simulink model "pdctrl"  (R2024b)
settings: Solver=VariableStepAuto  StartTime=0.0  StopTime=10.0  RelTol=1e-3
libraries: slpidlib x1
settings Model: Creator=Dell  LastModifiedBy=Dell

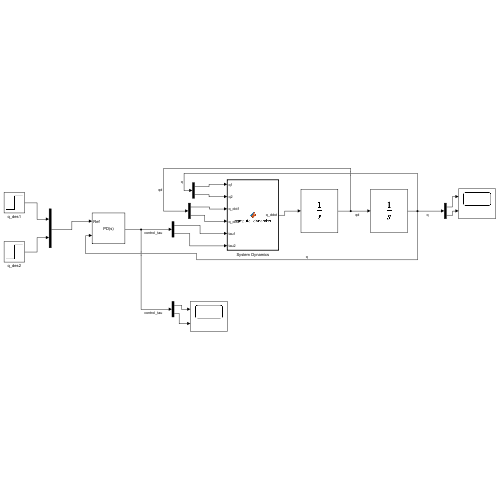
[thumbnail: Simulink's stored preview of the top-level diagram]
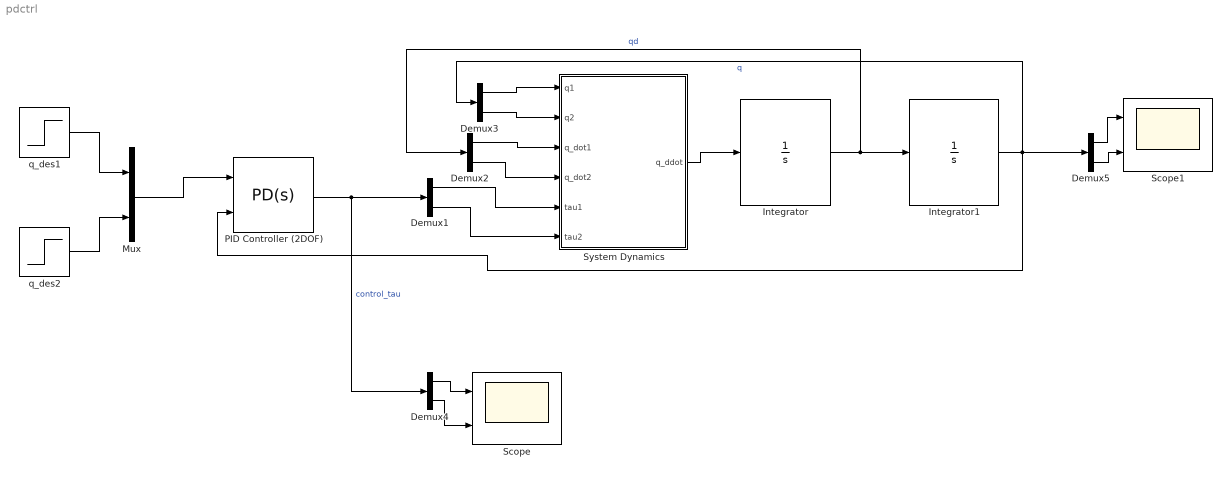
== system pdctrl ==
  Demux{1..5} (5 alike) : Demux  Outputs=2
  Integrator : Integrator  InitialCondition=[0;0]
  Integrator1 : Integrator  InitialCondition=[0, 0]
  Mux : Mux  Inputs=2
  PID Controller (2DOF) : slpidlib/PID Controller (2DOF)  Controller=PD  Form=Parallel  TimeDomain=Continuous-time  UseExternalTs=off  SampleTime=-1  IntegratorMethod=Forward Euler  FilterMethod=Forward Euler  ControllerParametersSource=internal  P=2000  I=0  UseKiTs=off  D=100  UseExternalDerivativeSource=off  N=100  UseFilter=on  b=1  c=1  TunerSelectOption=Transfer Function Based (PID Tuner App)  InitialConditionSource=internal  InitialConditionForIntegrator=0  InitialConditionForFilter=0  DifferentiatorICPrevScaledInput=0  ExternalReset=none  TrackingMode=off  Kt=1  LimitOutput=off  SatLimitsSource=internal  UpperSaturationLimit=inf  LowerSaturationLimit=-inf  LinearizeAsGain=on  AntiWindupMode=none  Kb=1  LimitIntegrator=off  UpperIntegratorSaturationLimit=inf  LowerIntegratorSaturationLimit=-inf  POutMin=[]  POutMax=[]  IOutMin=[]  IOutMax=[]  DOutMin=[]  DOutMax=[]  NOutMin=[]  NOutMax=[]  bOutMin=[]  bOutMax=[]  cOutMin=[]  cOutMax=[]  SumOutMin=[]  SumOutMax=[]  SaturationOutMin=[]  SaturationOutMax=[]  PParamMin=[]  PParamMax=[]  IParamMin=[]  IParamMax=[]  DParamMin=[]  DParamMax=[]  NParamMin=[]  NParamMax=[]  bParamMin=[]  bParamMax=[]  cParamMin=[]  cParamMax=[]  KbParamMin=[]  KbParamMax=[]  KtParamMin=[]  KtParamMax=[]  KbOutMin=[]  KbOutMax=[]  KtOutMin=[]  KtOutMax=[]  IntegratorOutMin=[]  IntegratorOutMax=[]  FilterOutMin=[]  FilterOutMax=[]  SumI1OutMin=[]  SumI1OutMax=[]  SumI2OutMin=[]  SumI2OutMax=[]  SumI3OutMin=[]  SumI3OutMax=[]  SumI4OutMin=[]  SumI4OutMax=[]  SumDOutMin=[]  SumDOutMax=[]  Sum1OutMin=[]  Sum1OutMax=[]  Sum2OutMin=[]  Sum2OutMax=[]  Sum3OutMin=[]  Sum3OutMax=[]  DifferentiatorOutMin=[]  DifferentiatorOutMax=[]  FilterDiffOutCoefMin=[]  FilterDiffOutCoefMax=[]  ReciprocalOutMin=[]  ReciprocalOutMax=[]  SumDenOutMin=[]  SumDenOutMax=[]  SumNumOutMin=[]  SumNumOutMax=[]  DivideOutMin=[]  DivideOutMax=[]  UdiffTsProdOutMin=[]  UdiffTsProdOutMax=[]  NTsProdOutMin=[]  NTsProdOutMax=[]  UintegralTsProdOutMin=[]  UintegralTsProdOutMax=[]  UngainTsProdOutMin=[]  UngainTsProdOutMax=[]  ClampingZeroOutDataTypeStr=Inherit: Inherit via back propagation  ClampingZeroOutMin=[]  ClampingZeroOutMax=[]  FilterDenConstantOutDataTypeStr=Inherit: Inherit via back propagation  FilterDenConstantOutMin=[]  FilterDenConstantOutMax=[]  PCopyOutDataTypeStr=Inherit: Inherit via back propagation  PCopyOutMin=[]  PCopyOutMax=[]  NCopyOutDataTypeStr=Inherit: Inherit via back propagation  NCopyOutMin=[]  NCopyOutMax=[]  IntegratorContinuousStateAttributes=''  IntegratorStateMustResolveToSignalObject=off  IntegratorRTWStateStorageClass=Auto  FilterContinuousStateAttributes=''  FilterStateMustResolveToSignalObject=off  FilterRTWStateStorageClass=Auto  ParallelPVariant=InternalParameters  IdealPVariant=Disabled  IVariant=Disabled  DVariant=InternalParameters  bVariant=InternalParameters  cVariant=InternalParameters  IntegratorVariant=Disabled  SatVariant=Disabled  AWVariant=Disabled  PCopyVariant=Disabled  TRVariant=Disabled  FdbkBlocksVariant=Forward  IdealPFdbkVariant=Disabled  SatFdbkVariant=Disabled  DerivativeFilterVariant=ContFilter  NVariant=InternalParameters  NCopyVariant=Disabled  FilterICVariant=InternalICsFilter  IntegratorICVariant=Disabled  ExternalResetVariant=Disabled  TRSumVariant=Passthrough  SumFdbkVariant=Disabled  SumVariant=Sum_PD  TsampFilterVariant=InternalTs  TsampNgainVariant=Passthrough  TsampIntegralVariant=Disabled_SignalSpec  ExternalSaturationOutDataTypeStr=Inherit: Same as second input  DerivativeSourceVariant=ErrorSignal  PreIntVariant=InternalPreInt
  Scope : Scope  NumInputPorts=2
  Scope1 : Scope  NumInputPorts=2
  System Dynamics : MATLAB Function  TreatAsAtomicUnit=on
  q_des1 : Step  Time=0  After=1.0472  SampleTime=0
  q_des2 : Step  Time=0  After=1.5708  SampleTime=0
  wires:
  Integrator/1 -> Integrator1/1, Demux2/1  "qd"
  System Dynamics/1(q_ddot) -> Integrator/1
  PID Controller (2DOF)/1 -> Demux4/1, Demux1/1  "control_tau"
  Integrator1/1 -> Demux5/1, Demux3/1, PID Controller (2DOF)/2  "q"
  Mux/1 -> PID Controller (2DOF)/1
  q_des1/1 -> Mux/1
  q_des2/1 -> Mux/2
  Demux1/1 -> System Dynamics/5(tau1)
  Demux1/2 -> System Dynamics/6(tau2)
  Demux2/1 -> System Dynamics/3(q_dot1)
  Demux2/2 -> System Dynamics/4(q_dot2)
  Demux3/1 -> System Dynamics/1(q1)
  Demux3/2 -> System Dynamics/2(q2)
  Demux4/1 -> Scope/1
  Demux4/2 -> Scope/2
  Demux5/1 -> Scope1/1
  Demux5/2 -> Scope1/2

== matlab function pdctrl/System Dynamics ==
  data: q1 input; q2 input; q_dot1 input; q_ddot output; q_dot2 input; tau1 input; tau2 input
function q_ddot = compute_dynamics(q1, q2, q_dot1, q_dot2, tau1, tau2)
    % Define system parameters inside the function
    m1 = 1;
    I1 = 0.12;
    me = 2;
    delta_e = 30 * pi/180; % Convert to radians
    lc1 = 0.5;
    le = 0.25;
    lcc = 0.6;

    % Compute system coefficients
    a1 = I1 + m1*lc1^2 + le + me*lcc^2 + me*lc1^2;
    a2 = le + me*lcc^2;
    a3 = me*lc1*lcc*cos(delta_e);
    a4 = me*lc1*lcc*sin(delta_e);

    % Compute Mass Matrix H(q)
    H = [a1 + 2*a3*cos(q2) + 2*a4*sin(q2), a2 + a3*cos(q2) + a4*sin(q2);
         a2 + a3*cos(q2) + a4*sin(q2), a2];

    % Compute Coriolis and Centripetal Matrix C(q, q_dot)
    h = a3*sin(q2) - a4*cos(q2);
    C = [-h*q_dot2, -h*(q_dot1 + q_dot2);
          h*q_dot1, 0];

    % Compute joint accelerations
    q_ddot = H \ ([tau1; tau2] - C * [q_dot1; q_dot2]);
end
